simulink model "Peregrine_Falcon_Model"  (R2025a)
settings: Solver=VariableStepAuto  StartTime=0.0  StopTime=2.5  RelTol=1e-3
undefined symbols (not defined in the file): A1, A2, Cd1, Cd2, g, m, rho

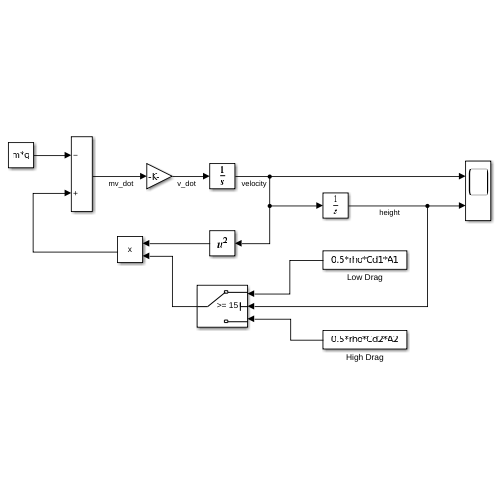
[thumbnail: Simulink's stored preview of the top-level diagram]
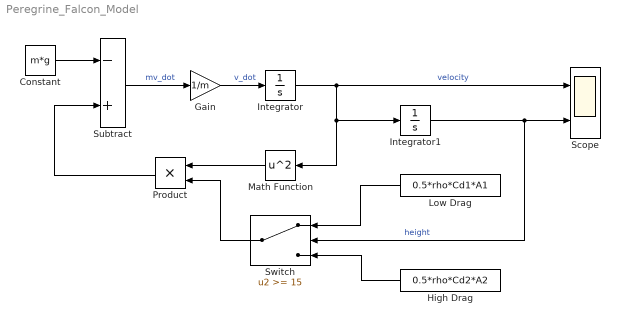
== system Peregrine_Falcon_Model ==
  Constant : Constant  Value=m*g
  Gain : Gain  Gain=1/m
  High Drag : Constant  Value=0.5*rho*Cd2*A2
  Integrator : Integrator  InitialCondition=-10
  Integrator1 : Integrator  InitialCondition=60
  Low Drag : Constant  Value=0.5*rho*Cd1*A1
  Math Function : Math  Operator=square
  Product : Product
  Scope : Scope  NumInputPorts=2
      settings: ActiveDisplayYMinimum=-32.260176872366394  ActiveDisplayYMaximum=70.251130763596265
  Subtract : Sum  Inputs=-+
  Switch : Switch  Threshold=15  SaturateOnIntegerOverflow=off  InputSameDT=off
  wires:
  Constant/1 -> Subtract/1
  Subtract/1 -> Gain/1  "mv_dot"
  Gain/1 -> Integrator/1  "v_dot"
  Integrator/1 -> Scope/1, Integrator1/1, Math Function/1  "velocity"
  Math Function/1 -> Product/1
  Product/1 -> Subtract/2
  Switch/1 -> Product/2
  Integrator1/1 -> Switch/2, Scope/2  "height"
  Low Drag/1 -> Switch/1
  High Drag/1 -> Switch/3
